simulink model "MultirotorSimArduCopter"  (R2015b)
settings: Solver=ode45  SolverMode=SingleTasking  StartTime=0.0  StopTime=100  MaxStep=Simulation.TS_MAX  RelTol=1e-6
InitFcn:
  | OldInitializeParameters
StopFcn:
  | %sim_complete_dlg
undefined symbols (not defined in the file or in its folder): b, batt_volt_nom, beta, Cd, Cdm, G, I, I_R, init_eta, init_M, init_nu_B, init_xi, init_xi_d1, k, K_e, K_T, l, m, R, rhoAir
libraries: simulink_extras x5
settings Model: Creator=zche092  LastModifiedBy=jeremie
settings DataIOCC: LimitDataPoints=off  SaveFormat=Array  SaveOutput=off  DSMLogging=off  VisualizeSimOutput=off  SaveTime=off  OutputOption=SpecifiedOutputTimes  OutputTimes=tSim
settings OptimizationCC: BlockReduction=off  BooleanDataType=off
settings DebuggingCC: SaveWithParameterizedLinksMsg=none  UnderspecifiedInitializationDetection=Classic  MergeDetectMultiDrivingBlocksExec=none  SignalResolutionControl=TryResolveAllWithWarning
settings HardwareCC: ProdBitPerPointer=32  ProdLargestAtomicFloat=None  ProdIntDivRoundTo=Undefined  ProdEndianess=Unspecified  ProdWordSize=32  ProdHWDeviceType=32-bit Generic  TargetUnknown=on
settings GRTTargetCC: GeneratePreprocessorConditionals=Disable all
settings ConfigComp: CovModelRefEnable=Off  CovSFcnEnable=off

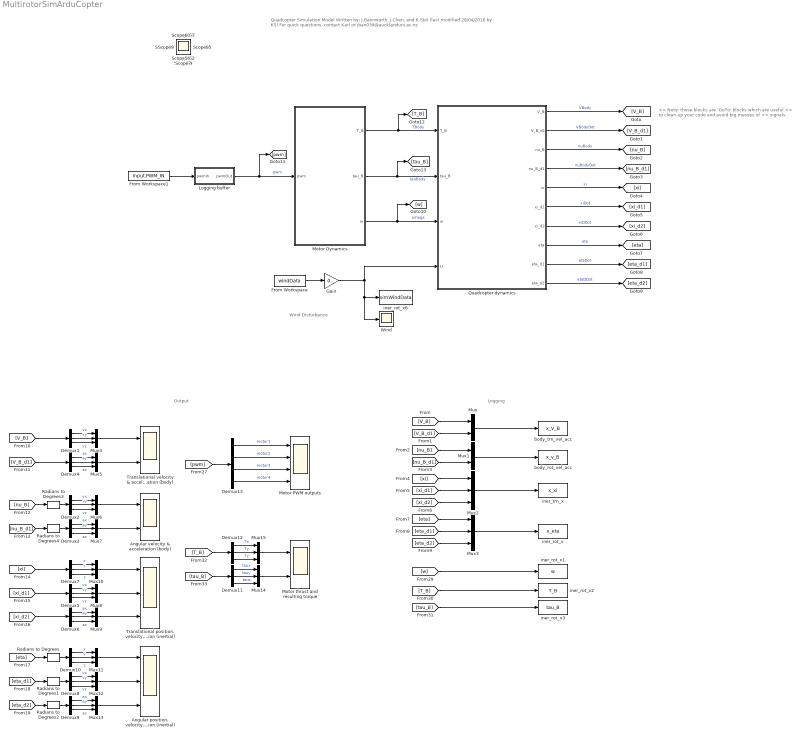
== system MultirotorSimArduCopter ==
  note: << Note: those blocks are 'GoTo' blocks which are useful
      | << to clean-up your code and avoid big messes of
      | << signals.
  note: Output
  note: Logging
  note: Wind Disturbance
  note: Quadcopter Simulation Model
      |
      | Written by: J.Bannwarth, J.Chen, and K.Stol (last modified 28/04/2016 by KS)
      | For quick questions, contact Karl or jban039@aucklanduni.ac.nz
  "Angular position, velocity, & acceleration (inertial)" : Scope  NumInputPorts=3
  Angular velocity & acceleration (body) : Scope  NumInputPorts=2
  Demux{1..12} (12 alike) : Demux  Outputs=3
  Demux13 : Demux
  From Workspace : FromWorkspace  VariableName=windData  SampleTime=0
  From Workspace1 : FromWorkspace  VariableName=Input.PWM_IN  SampleTime=0
  Gain : Gain  Gain=0
  Logging buffer : Subsystem
  Motor Dynamics : Subsystem
  Motor PWM outputs : Scope  NumInputPorts=4
  Motor thrust and resulting torque : Scope  NumInputPorts=2
  Mux : Mux  Inputs=2
  Mux1 : Mux  Inputs=2
  Mux{2..15} (14 alike) : Mux  Inputs=3
  Quadcopter dynamics : Subsystem
  Radians to Degrees{,1..4} (5 alike) : simulink_extras/Transformations/Radians to Degrees
  "Translational position, velocity, & acceleration (inertial)" : Scope  NumInputPorts=3
  Translational velocity & acceleration (body) : Scope  NumInputPorts=2
  Wind : Scope
  body_rot_vel_acc : ToWorkspace  VariableName=x_v_B  SampleTime=-1
  body_trn_vel_acc : ToWorkspace  VariableName=x_V_B  SampleTime=-1
  iner_rot_x : ToWorkspace  VariableName=x_eta  SampleTime=-1
  iner_rot_x1 : ToWorkspace  VariableName=w  SampleTime=-1
  iner_rot_x2 : ToWorkspace  VariableName=T_B  SampleTime=-1
  iner_rot_x3 : ToWorkspace  VariableName=tau_B  SampleTime=-1
  iner_rot_x6 : ToWorkspace  VariableName=simWindData  SampleTime=-1
  iner_trn_x : ToWorkspace  VariableName=x_xi  SampleTime=-1
  Scope{,1..60} (61 alike) : Scope
  wires:
  Mux/1 -> body_trn_vel_acc/1
  Motor Dynamics/1(T_B) -> [T_B], Quadcopter dynamics/1(T_B)  "TBody"
  Motor Dynamics/2(tau_B) -> [tau_B], Quadcopter dynamics/2(tau_B)  "tauBody"
  Quadcopter dynamics/1(V_B) -> [V_B]  "VBody"
  Quadcopter dynamics/9(eta_d1) -> [eta_d1]  "etaDot"
  Quadcopter dynamics/2(V_B_d1) -> [V_B_d1]  "VBodyDot"
  Quadcopter dynamics/6(xi_d1) -> [xi_d1]  "xiDot"
  Quadcopter dynamics/3(nu_B) -> [nu_B]  "nuBody"
  Quadcopter dynamics/4(nu_B_d1) -> [nu_B_d1]  "nuBodyDot"
  Quadcopter dynamics/10(eta_d2) -> [eta_d2]  "etaDDot"
  Quadcopter dynamics/8(eta) -> [eta]  "eta"
  Quadcopter dynamics/7(xi_d2) -> [xi_d2]  "xiDDot"
  Quadcopter dynamics/5(xi) -> [xi]  "xi"
  Mux1/1 -> body_rot_vel_acc/1
  Mux3/1 -> iner_rot_x/1
  [eta_d1] -> Mux3/2
  [eta] -> Mux3/1
  [eta_d2] -> Mux3/3
  [xi_d1] -> Mux2/2
  [xi] -> Mux2/1
  [xi_d2] -> Mux2/3
  [nu_B_d1] -> Mux1/2
  [nu_B] -> Mux1/1
  [V_B_d1] -> Mux/2
  [V_B] -> Mux/1
  Mux2/1 -> iner_trn_x/1
  [V_B] -> Demux1/1
  [V_B_d1] -> Demux4/1
  [xi] -> Demux7/1
  [xi_d2] -> Demux6/1
  [xi_d1] -> Demux5/1
  [eta] -> Radians to Degrees/1
  [eta_d1] -> Radians to Degrees1/1
  [eta_d2] -> Radians to Degrees2/1
  Gain/1 -> Wind/1, iner_rot_x6/1, Quadcopter dynamics/4(U)
  From Workspace/1 -> Gain/1
  Mux4/1 -> Translational velocity & acceleration (body)/1
  Mux5/1 -> Translational velocity & acceleration (body)/2
  [nu_B] -> Radians to Degrees3/1
  [nu_B_d1] -> Radians to Degrees4/1
  Demux2/3 -> Mux6/3  "vz"
  Demux2/2 -> Mux6/2  "vy"
  Demux2/1 -> Mux6/1  "vx"
  Mux6/1 -> Angular velocity & acceleration (body)/1
  Demux3/3 -> Mux7/3  "az"
  Demux3/2 -> Mux7/2  "ay"
  Demux3/1 -> Mux7/1  "ax"
  Mux7/1 -> Angular velocity & acceleration (body)/2
  Demux1/3 -> Mux4/3  "vz"
  Demux1/2 -> Mux4/2  "vy"
  Demux1/1 -> Mux4/1  "vx"
  Demux4/3 -> Mux5/3  "az"
  Demux4/2 -> Mux5/2  "ay"
  Demux4/1 -> Mux5/1  "ax"
  Demux5/3 -> Mux8/3  "vz"
  Demux5/2 -> Mux8/2  "vy"
  Demux5/1 -> Mux8/1  "vx"
  Demux6/3 -> Mux9/3  "az"
  Demux6/2 -> Mux9/2  "ay"
  Demux6/1 -> Mux9/1  "ax"
  Demux7/3 -> Mux10/3  "z"
  Demux7/2 -> Mux10/2  "y"
  Demux7/1 -> Mux10/1  "x"
  Mux8/1 -> "Translational position, velocity, & acceleration (inertial)"/2
  Mux10/1 -> "Translational position, velocity, & acceleration (inertial)"/1
  Mux9/1 -> "Translational position, velocity, & acceleration (inertial)"/3
  Radians to Degrees/1 -> Demux10/1
  Radians to Degrees2/1 -> Demux9/1
  Radians to Degrees1/1 -> Demux8/1
  Demux8/3 -> Mux12/3  "vz"
  Demux8/2 -> Mux12/2  "vy"
  Demux8/1 -> Mux12/1  "vx"
  Demux9/3 -> Mux13/3  "az"
  Demux9/2 -> Mux13/2  "ay"
  Demux9/1 -> Mux13/1  "ax"
  Demux10/3 -> Mux11/3  "z"
  Demux10/2 -> Mux11/2  "y"
  Demux10/1 -> Mux11/1  "x"
  Mux12/1 -> "Angular position, velocity, & acceleration (inertial)"/2
  Mux11/1 -> "Angular position, velocity, & acceleration (inertial)"/1
  Mux13/1 -> "Angular position, velocity, & acceleration (inertial)"/3
  Radians to Degrees4/1 -> Demux3/1
  Radians to Degrees3/1 -> Demux2/1
  Demux11/3 -> Mux14/3  "tauz"
  Demux11/2 -> Mux14/2  "tauy"
  Demux11/1 -> Mux14/1  "taux"
  Mux14/1 -> Motor thrust and resulting torque/2
  Demux12/3 -> Mux15/3  "Tz"
  Demux12/2 -> Mux15/2  "Ty"
  Demux12/1 -> Mux15/1  "Tx"
  Mux15/1 -> Motor thrust and resulting torque/1
  Motor Dynamics/3(w) -> [w], Quadcopter dynamics/3(w)  "omega"
  From Workspace1/1 -> Logging buffer/1(pwmIn)
  Demux13/4 -> Motor PWM outputs/4  "motor4"
  Demux13/1 -> Motor PWM outputs/1  "motor1"
  Demux13/2 -> Motor PWM outputs/2  "motor2"
  Demux13/3 -> Motor PWM outputs/3  "motor3"
  [w] -> iner_rot_x1/1
  [T_B] -> iner_rot_x2/1
  [tau_B] -> iner_rot_x3/1
  [tau_B] -> Demux11/1
  [T_B] -> Demux12/1
  [pwm] -> Demux13/1
  Logging buffer/1(pwmOut) -> [pwm], Motor Dynamics/1(pwm)  "pwm"

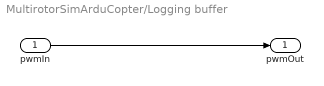
== system MultirotorSimArduCopter/Logging buffer ==
  pwmIn : Inport
  pwmOut : Outport
  wires:
  pwmIn/1 -> pwmOut/1

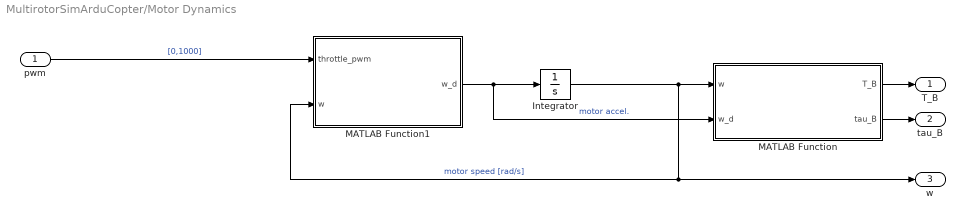
== system MultirotorSimArduCopter/Motor Dynamics ==
  pwm : Inport
  Integrator : Integrator  InitialCondition=init_M
  MATLAB Function : MATLAB Function  TreatAsAtomicUnit=on
  MATLAB Function1 : MATLAB Function  TreatAsAtomicUnit=on
  T_B : Outport
  tau_B : Outport  Port=2
  w : Outport  Port=3
  wires:
  MATLAB Function1/1(w_d) -> MATLAB Function/2(w_d), Integrator/1  "motor accel."
  MATLAB Function/2(tau_B) -> tau_B/1
  MATLAB Function/1(T_B) -> T_B/1
  Integrator/1 -> MATLAB Function/1(w), w/1, MATLAB Function1/2(w)  "motor speed [rad/s]"
  pwm/1 -> MATLAB Function1/1(throttle_pwm)  "[0,1000]"

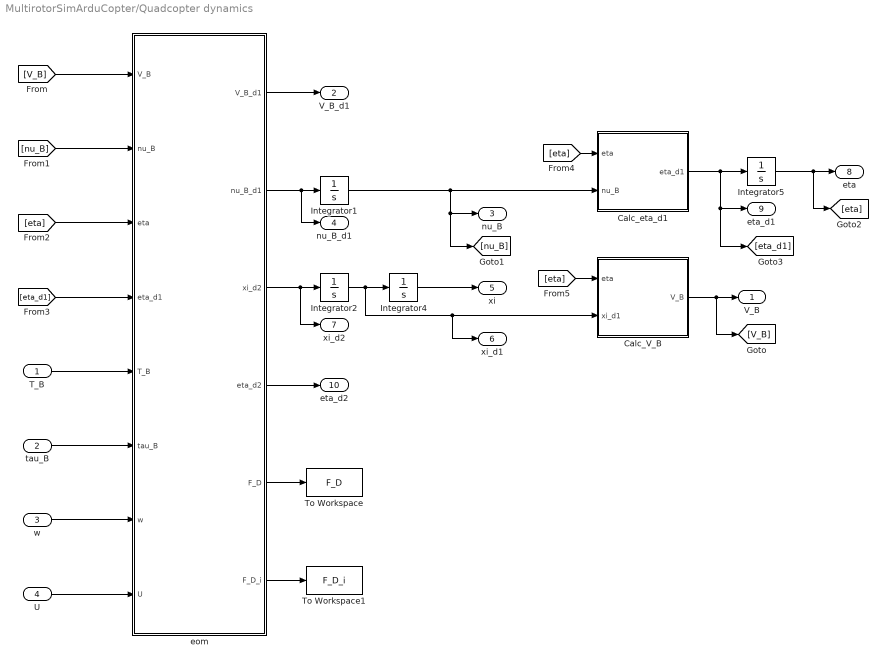
== system MultirotorSimArduCopter/Quadcopter dynamics ==
  T_B : Inport
  tau_B : Inport  Port=2
  w : Inport  Port=3
  U : Inport  Port=4
  Calc_V_B : MATLAB Function  TreatAsAtomicUnit=on
  Calc_eta_d1 : MATLAB Function  TreatAsAtomicUnit=on
  Integrator1 : Integrator  InitialCondition=init_nu_B
  Integrator2 : Integrator  InitialCondition=init_xi_d1
  Integrator4 : Integrator  InitialCondition=init_xi
  Integrator5 : Integrator  InitialCondition=init_eta  WrapState=on
  To Workspace : ToWorkspace  VariableName=F_D  SampleTime=-1
  To Workspace1 : ToWorkspace  VariableName=F_D_i  SampleTime=-1
  eom : MATLAB Function  TreatAsAtomicUnit=on
  V_B : Outport
  V_B_d1 : Outport  Port=2
  nu_B : Outport  Port=3
  nu_B_d1 : Outport  Port=4
  xi : Outport  Port=5
  xi_d1 : Outport  Port=6
  xi_d2 : Outport  Port=7
  eta : Outport  Port=8
  eta_d1 : Outport  Port=9
  eta_d2 : Outport  Port=10
  wires:
  eom/1(V_B_d1) -> V_B_d1/1
  eom/2(nu_B_d1) -> Integrator1/1, nu_B_d1/1
  Integrator2/1 -> xi_d1/1, Calc_V_B/2(xi_d1), Integrator4/1
  Integrator1/1 -> [nu_B], nu_B/1, Calc_eta_d1/2(nu_B)
  Integrator4/1 -> xi/1
  [nu_B] -> eom/2(nu_B)
  [V_B] -> eom/1(V_B)
  Integrator5/1 -> eta/1, [eta]
  [eta] -> eom/3(eta)
  [eta_d1] -> eom/4(eta_d1)
  w/1 -> eom/7(w)
  tau_B/1 -> eom/6(tau_B)
  T_B/1 -> eom/5(T_B)
  eom/3(xi_d2) -> Integrator2/1, xi_d2/1
  eom/4(eta_d2) -> eta_d2/1
  eom/5(F_D) -> To Workspace/1
  U/1 -> eom/8(U)
  eom/6(F_D_i) -> To Workspace1/1
  Calc_eta_d1/1(eta_d1) -> [eta_d1], eta_d1/1, Integrator5/1
  [eta] -> Calc_eta_d1/1(eta)
  Calc_V_B/1(V_B) -> [V_B], V_B/1
  [eta] -> Calc_V_B/1(eta)

== matlab function MultirotorSimArduCopter/Quadcopter dynamics/eom ==
  data: V_B input; V_B_d1 output; nu_B input; eta input; eta_d1 input; T_B input; tau_B input; w input; U input; m parameter; nu_B_d1 output; I parameter; I_R parameter; Cd parameter; Cdm parameter; rhoAir parameter; G parameter; xi_d2 output; eta_d2 output; F_D output; F_D_i output
function [V_B_d1,nu_B_d1,xi_d2,eta_d2,F_D,F_D_i] = fcn(V_B,nu_B,eta,eta_d1,T_B,tau_B,w,U, m,I,I_R,Cd,Cdm,rhoAir,G)
%#codegen

% Rotation matrices
Sphi = sin(eta(1));
Stheta = sin(eta(2));
Spsi = sin(eta(3));
Cphi = cos(eta(1));
Ctheta = cos(eta(2));
Cpsi = cos(eta(3));
Ttheta = tan(eta(2));
phi_d = eta_d1(1);
theta_d = eta_d1(2);

R = [Cpsi*Ctheta,   Cpsi*Stheta*Sphi-Spsi*Cphi, Cpsi*Stheta*Cphi+Spsi*Sphi;
	Spsi*Ctheta,    Spsi*Stheta*Sphi+Cpsi*Cphi, Spsi*Stheta*Cphi-Cpsi*Sphi;
	-Stheta,        Ctheta*Sphi,                Ctheta*Cphi+Spsi*Sphi];     % rotation matrix from body frame to inertial frame

dWInv = [0,    phi_d*Cphi*Ttheta+theta_d*Sphi/Ctheta^2,    -phi_d*Sphi*Ctheta+theta_d*Cphi/Ctheta^2;
          0,    -phi_d*Sphi,                                -phi_d*Cphi;
	      0,    phi_d*Cphi/Ctheta+phi_d*Sphi*Ttheta/Ctheta, -phi_d*Sphi/Ctheta+theta_d*Cphi*Ttheta/Ctheta];
      
WInv = [1, Sphi*Ttheta,    Cphi*Ttheta;
         0, Cphi,           -Sphi;
         0, Sphi/Ctheta,    Cphi/Ctheta];

% Gyroscopic moment
M_Gi = zeros(3,4);
for i=1:4
	% Angular momentum in motor frame
	H_Mi = I_R*[0;0;(-1)^i*w(i)];

	% Gyroscopic moment vectors in body frame
	M_Gi(:,i) = cross(nu_B,H_Mi);
end

M_G = sum(M_Gi,2);

% Drag force
R_U = [1,0,0;0,1,0;0,0,-1];     % Rotation matrix from Wind frame to Inertial frame 

% Apparent velocity
V_B_app = V_B + R'*R_U*U;
V_B_app_mag = norm(V_B_app);    % magnitude of apparent velocity

% Calculate drag force
F_D = 0.5*rhoAir*Cd*(V_B_app_mag.*V_B_app);    % drag force in Body frame
F_D_i = R*F_D;                              % drag force in Inertial frame

% Drag moment, applied to independent axes
M_D = 0.5*rhoAir*Cdm*norm(nu_B)*nu_B;

% Body frame accelerations
V_B_d1 = (1/m)*(R'*G+T_B-cross(nu_B,m*V_B)-F_D);
nu_B_d1 = I\(tau_B-cross(nu_B,I*nu_B)-M_G-M_D);

% Inertial frame accelerations
xi_d2 = (1/m)*(G+R*T_B - R*F_D);
eta_d2 = dWInv*nu_B + WInv*nu_B_d1;

% Check centripetal force in inertial frame
F_C = R*cross(nu_B,m*V_B);
end

== matlab function MultirotorSimArduCopter/Quadcopter dynamics/Calc_eta_d1 ==
  data: eta input; nu_B input; eta_d1 output
function eta_d1 = fcn(eta,nu_B)
%#codegen

Sphi = sin(eta(1));
Cphi = cos(eta(1));
Ctheta = cos(eta(2));
Ttheta = tan(eta(2));
      
WInv = [1, Sphi*Ttheta,    Cphi*Ttheta;
         0, Cphi,           -Sphi;
         0, Sphi/Ctheta,    Cphi/Ctheta];
     
eta_d1 = WInv*nu_B;

== matlab function MultirotorSimArduCopter/Quadcopter dynamics/Calc_V_B ==
  data: eta input; V_B output; xi_d1 input
function V_B = fcn(eta,xi_d1)
%#codegen

Sphi = sin(eta(1));
Stheta = sin(eta(2));
Spsi = sin(eta(3));
Cphi = cos(eta(1));
Ctheta = cos(eta(2));
Cpsi = cos(eta(3));

R = [Cpsi*Ctheta,   Cpsi*Stheta*Sphi-Spsi*Cphi, Cpsi*Stheta*Cphi+Spsi*Sphi;
	Spsi*Ctheta,    Spsi*Stheta*Sphi+Cpsi*Cphi, Spsi*Stheta*Cphi-Cpsi*Sphi;
	-Stheta,        Ctheta*Sphi,                Ctheta*Cphi+Spsi*Sphi];     % rotation matrix from body frame to inertial frame

V_B = R'*xi_d1;

== matlab function MultirotorSimArduCopter/Motor Dynamics/MATLAB Function ==
  data: w input; T_B output; w_d input; k parameter; b parameter; l parameter; beta parameter; tau_B output; I_R parameter
function [T_B,tau_B] = motor_force_torque(w,w_d, k,b,l,beta,I_R)
%#codegen

% Motor force/torque vectors in motor frame
ind_Mi = (-1).^((1:1:4));
T_Mi = [zeros(2,4); k*(w'.^2)];
tau_Mi = [zeros(2,4); (b*(w'.^2)+I_R(3,3)*w_d').*ind_Mi];

% Initialise matrices to store motor force/torque vectors
T_Bi = zeros(3,4);
tau_Bi = zeros(3,4);

% Calculate forces and moments from each motor in the body frame
for i=1:4
	% Matrix to calculate moments in body frame due to rotor thrust
 	R_F_B = [ 0,              0,              l*sin(beta(i)) ;
              0,              0,             -l*cos(beta(i)) ;
             -l*sin(beta(i)), l*cos(beta(i)), 0             ];

	% Motor force/torque vectors in body frame
	T_Bi(:,i) = T_Mi(:,i);
	tau_Bi(:,i) = tau_Mi(:,i)+R_F_B*T_Mi(:,i);
end

% Total force/torque in body frame
T_B = sum(T_Bi,2);
tau_B = sum(tau_Bi,2);

end

== matlab function MultirotorSimArduCopter/Motor Dynamics/MATLAB Function1 ==
  data: throttle_pwm input; w_d output double size=4; w input; batt_volt_nom parameter; K_T parameter; K_e parameter; R parameter; I_R parameter; b parameter
function w_d = fcn(throttle_pwm,w, batt_volt_nom,K_T,K_e,R,I_R,b)
%#codegen

v = throttle_pwm*batt_volt_nom/1000;    % applied motor voltages
current = (v - K_e*w)/R;      % motor current, ignoring inductance

net_torque = K_T*current - b*w.^2;

w_d = net_torque/I_R(3,3);  % motor angular acceleration
